simulink model "task_1_sim"  (R2023a)
settings: Solver=VariableStepAuto  StartTime=0.0  StopTime=5  MaxStep=1e-5  RelTol=1e-5
undefined symbols (not defined in the file): A, B, Bf, Cz, G, K1, K2, w_f0, x0
settings Model: Creator=user  LastModifiedBy=user

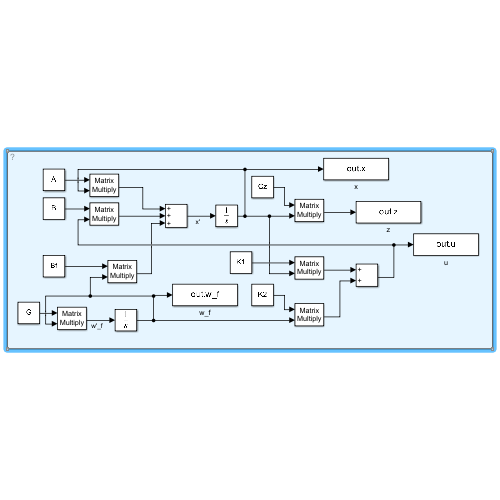
[thumbnail: Simulink's stored preview of the top-level diagram]
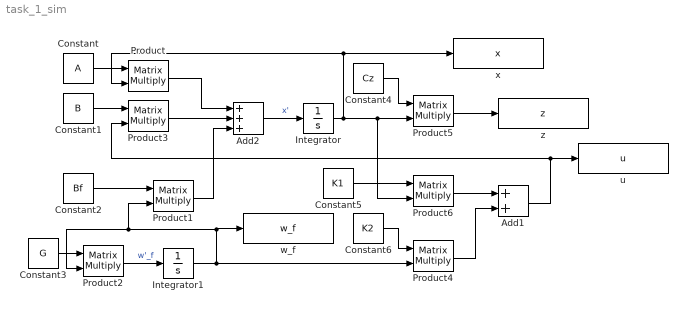
== system task_1_sim ==
  Add1 : Sum
  Add2 : Sum  Inputs=+++
  Constant : Constant  Value=A
  Constant1 : Constant  Value=B
  Constant2 : Constant  Value=Bf
  Constant3 : Constant  Value=G
  Constant4 : Constant  Value=Cz  VectorParams1D=off
  Constant5 : Constant  Value=K1  VectorParams1D=off
  Constant6 : Constant  Value=K2  VectorParams1D=off
  Integrator : Integrator  InitialCondition=x0
  Integrator1 : Integrator  InitialCondition=w_f0
  Product{,1..6} (7 alike) : Product  Multiplication=Matrix(*)
  u : ToWorkspace  VariableName=u  SaveFormat=Timeseries  SampleTime=-1
  w_f : ToWorkspace  VariableName=w_f  SaveFormat=Timeseries  SampleTime=-1
  x : ToWorkspace  VariableName=x  SaveFormat=Timeseries  SampleTime=-1
  z : ToWorkspace  VariableName=z  SaveFormat=Timeseries  SampleTime=-1
  wires:
  Constant/1 -> Product/1
  Integrator/1 -> Product5/2, Product6/2, x/1, Product/2
  Constant1/1 -> Product3/1
  Add1/1 -> Product3/2, u/1
  Product3/1 -> Add2/2
  Product/1 -> Add2/1
  Add2/1 -> Integrator/1  "x'"
  Constant2/1 -> Product1/1
  Integrator1/1 -> Product2/2, Product1/2, w_f/1, Product4/2
  Product1/1 -> Add2/3
  Product5/1 -> z/1
  Constant4/1 -> Product5/1
  Constant3/1 -> Product2/1
  Product2/1 -> Integrator1/1  "w'_f"
  Constant5/1 -> Product6/1
  Constant6/1 -> Product4/1
  Product6/1 -> Add1/1
  Product4/1 -> Add1/2
